simulink model "RLC_Simulink"  (R2023b)
settings: Solver=VariableStepAuto  StartTime=0.0  StopTime=0.002  RelTol=1e-3
values from neighbouring files (symbols this model uses):
  C = 0.1e-6    (= 1e-07)    [RLC.m]
  L = 4e-3    (= 0.004)    [RLC.m]
  R = 100    [RLC.m]
settings Model: Creator=andre  LastModifiedBy=andre

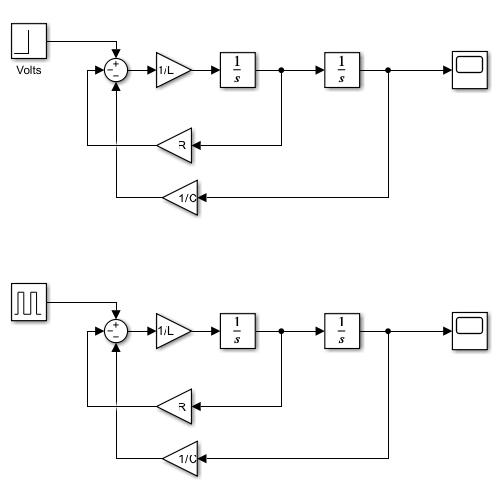
[thumbnail: Simulink's stored preview of the top-level diagram]
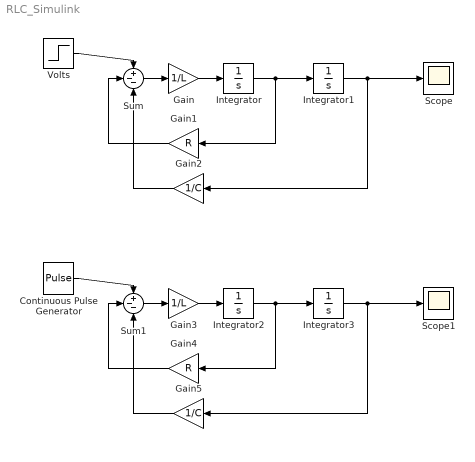
== system RLC_Simulink ==
  Continuous Pulse Generator : DiscretePulseGenerator  PulseType=Time based  Amplitude=12  Period=0.002  PulseWidth=50
  Gain : Gain  Gain=1/L
  Gain1 : Gain  Gain=R
  Gain2 : Gain  Gain=1/C
  Gain3 : Gain  Gain=1/L
  Gain4 : Gain  Gain=R
  Gain5 : Gain  Gain=1/C
  Integrator{,1..3} (4 alike) : Integrator
  Scope : Scope
  Scope1 : Scope
  Sum : Sum  Inputs=+--
  Sum1 : Sum  Inputs=+--
  Volts : Step  Time=0  After=12  SampleTime=0
  wires:
  Integrator/1 -> Gain1/1, Integrator1/1
  Sum/1 -> Gain/1
  Gain/1 -> Integrator/1
  Gain1/1 -> Sum/2
  Integrator1/1 -> Scope/1, Gain2/1
  Gain2/1 -> Sum/3
  Volts/1 -> Sum/1
  Integrator2/1 -> Gain4/1, Integrator3/1
  Sum1/1 -> Gain3/1
  Integrator3/1 -> Scope1/1, Gain5/1
  Gain4/1 -> Sum1/2
  Gain5/1 -> Sum1/3
  Gain3/1 -> Integrator2/1
  Continuous Pulse Generator/1 -> Sum1/1
